simulink model "et_robocon_dev_guy_arch"  (R2013b)
settings: Solver=FixedStepDiscrete  SolverMode=SingleTasking  StartTime=0.0  StopTime=inf  FixedStep=balancer_ts  RelTol=1e-3
undefined symbols (not defined in the file): a_d, a_r, balancerStates_Bus0, Batt, battery_gain, battery_offset, cmd_max, current_mode_status, current_task_operation_status, DiscIntNeverNeededParam, exec_period, Init_Bus0, K, k_f, k_i, k_phidot, k_thetadot, lightCalib, phi_des, R, STATE, TRACK_MODE_LIST, ts2, W
libraries: legonxtlib x34, simulink x19, simulink_extras x4
(part 2 of 5)

== system et_robocon_dev_guy_arch/Main Controller/normal_operation_modes.line_tracking_after_seesaw/line_tracking_mode.tail_controller ==
  note: Could be improved, PI for example
  current : Inport  OutDataTypeStr=single  PortDimensions=1
  desired : Inport  Port=2  OutDataTypeStr=single  PortDimensions=1
  f : TriggerPort  TriggerType=function-call
      settings: CopyFcn=Stateflow.SLINSF.SimulinkMan.removeBlockPreDeleteFcn  PreDeleteFcn=Stateflow.SLINSF.SimulinkMan.unsafePredeleteFcn
  Gain : Gain  Gain=250
  Saturation : Saturate  UpperLimit=100  LowerLimit=-100  OutDataTypeStr=single
  Sum : Sum  Inputs=|+-
  cmd : Outport  OutDataTypeStr=single  PortDimensions=1  InitialOutput=0
  wires:
  Sum/1 -> Gain/1
  current/1 -> Sum/2
  desired/1 -> Sum/1
  Gain/1 -> Saturation/1
  Saturation/1 -> cmd/1

== system et_robocon_dev_guy_arch/Main Controller/normal_operation_modes.line_tracking_after_seesaw/line_tracking_mode.turnLightOn ==
  f : TriggerPort  TriggerType=function-call
      settings: CopyFcn=Stateflow.SLINSF.SimulinkMan.removeBlockPreDeleteFcn  PreDeleteFcn=Stateflow.SLINSF.SimulinkMan.unsafePredeleteFcn
  Light Sensor Switch ON : S-Function  FunctionName=sfun_light_sw  Parameters=-1,ip,sw  EnableBusSupport=off  mask(Light Sensor ON/OFF Switch){ip=S3, sw=ON}
      mask prompts: ip "port:"; sw "switch"
      mask help: LEGO Mindstorms NXT Light Sensor switch.
      mask init:
      | [data, map]=imread('LIGHT_SENSOR.gif');
      | pic=ind2rgb(data,map);
      mask TypeOptions ip: S1 | S2 | S3 | S4
      mask TypeOptions sw: ON | OFF
      mask Display:
      | image(pic)
      | color('red')
      | fprintf('%s, %s',ip,sw)

== system et_robocon_dev_guy_arch/Main Controller/normal_operation_modes.line_tracking_mode/line_tracking_mode.Speak ==
  f : TriggerPort  TriggerType=function-call
      settings: CopyFcn=Stateflow.SLINSF.SimulinkMan.removeBlockPreDeleteFcn  PreDeleteFcn=Stateflow.SLINSF.SimulinkMan.unsafePredeleteFcn
  Constant : Constant  Value=50
  Speaker : legonxtlib/Speaker  sinputMode=Volume only  sspeakerFreq=800  sspeakerVolume=50  sspeakerDuration=100
  wires:
  Constant/1 -> Speaker/1

== system et_robocon_dev_guy_arch/Main Controller/normal_operation_modes.line_tracking_mode/line_tracking_mode.Track.analyzeEncoders ==
  rawSensors : Inport  OutDataTypeStr=Bus: Sensors_Bus  PortDimensions=1
  f : TriggerPort  TriggerType=function-call
      settings: CopyFcn=Stateflow.SLINSF.SimulinkMan.removeBlockPreDeleteFcn  PreDeleteFcn=Stateflow.SLINSF.SimulinkMan.unsafePredeleteFcn
  AngleCounter : Subsystem
  Bus Creator : BusCreator  Inputs=2
  Bus Selector : BusSelector  OutputSignals=theta_R,theta_L
  Signal Conversion : SignalConversion
  Signal Conversion1 : SignalConversion
  AngleCount : Outport  OutDataTypeStr=uint8  PortDimensions=1  InitialOutput=0
  EncoderReset : Outport  Port=2  OutDataTypeStr=single  PortDimensions=1  InitialOutput=0
  Angle : Outport  Port=3  OutDataTypeStr=single  PortDimensions=1  InitialOutput=0
  Distance : Outport  Port=4  OutDataTypeStr=single  PortDimensions=1  InitialOutput=0
  wires:
  rawSensors/1 -> Bus Selector/1
  Bus Creator/1 -> AngleCounter/1(EC)
  Bus Selector/1 -> Signal Conversion/1  "<theta_R>"
  Bus Selector/2 -> Signal Conversion1/1  "<theta_L>"
  Signal Conversion/1 -> Bus Creator/1  "R"
  Signal Conversion1/1 -> Bus Creator/2  "L"
  AngleCounter/1(AngleCount) -> AngleCount/1
  AngleCounter/2(EncoderReseted) -> EncoderReset/1
  AngleCounter/3(Angle) -> Angle/1
  AngleCounter/4(Distance) -> Distance/1

== system et_robocon_dev_guy_arch/Main Controller/normal_operation_modes.line_tracking_mode/line_tracking_mode.Track.lineTracker ==
  lightSignal : Inport  OutDataTypeStr=single  PortDimensions=1
  flagSteering : Inport  Port=2  OutDataTypeStr=single  PortDimensions=1
  PID : Inport  Port=3  OutDataTypeStr=single  PortDimensions=5
  fwd : Inport  Port=4  OutDataTypeStr=single  PortDimensions=1
  f : TriggerPort  TriggerType=function-call
      settings: CopyFcn=Stateflow.SLINSF.SimulinkMan.removeBlockPreDeleteFcn  PreDeleteFcn=Stateflow.SLINSF.SimulinkMan.unsafePredeleteFcn
  Gain : Gain  Gain=100
  Handler : Subsystem
  LCD : legonxtlib/LCD  slcdStr=PID  slcdLine=6  slcdFormat=Decimal
  Signal Conversion : SignalConversion
  SwitchForFreeSteering : Subsystem
  cmd : Outport  InitialOutput=[0 0]
  wires:
  Handler/1(cmd) -> Signal Conversion/1
  lightSignal/1 -> SwitchForFreeSteering/3(LightSens)
  SwitchForFreeSteering/1(Steering) -> Gain/1, Handler/1(steering)
  flagSteering/1 -> SwitchForFreeSteering/1(FlagSteering)
  PID/1 -> SwitchForFreeSteering/2(PID)
  fwd/1 -> Handler/2(fwd)
  Signal Conversion/1 -> cmd/1
  Gain/1 -> LCD/1

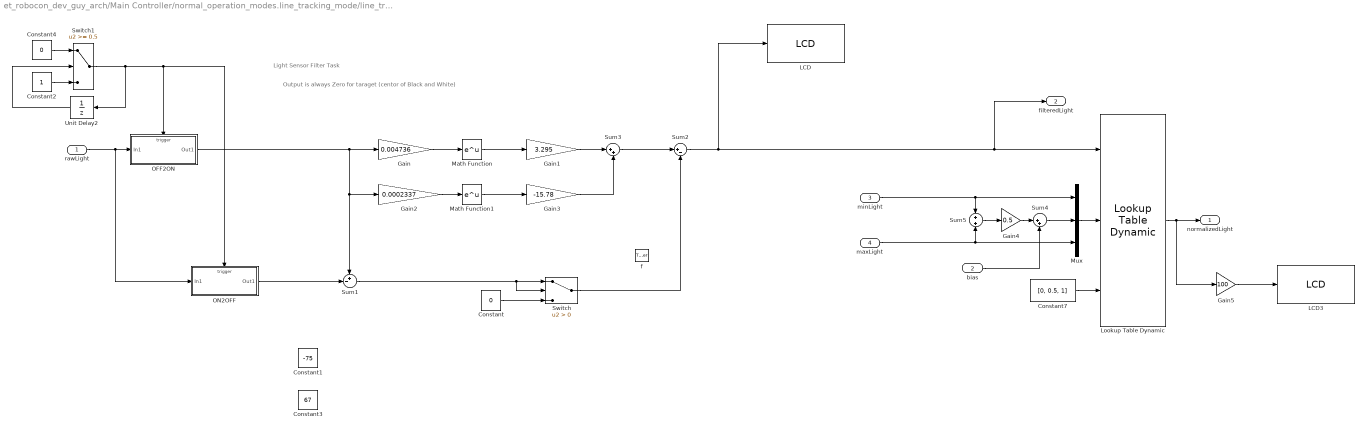
== system et_robocon_dev_guy_arch/Main Controller/normal_operation_modes.line_tracking_mode/line_tracking_mode.Track.processLight ==
  note: Output is always Zero for taraget (centor of Black and White)
  note: Light Sensor Filter Task
  rawLight : Inport  OutDataTypeStr=single  PortDimensions=1
  bias : Inport  Port=2  OutDataTypeStr=single  PortDimensions=1
  minLight : Inport  Port=3  OutDataTypeStr=single  PortDimensions=1
  maxLight : Inport  Port=4  OutDataTypeStr=single  PortDimensions=1
  f : TriggerPort  TriggerType=function-call
      settings: CopyFcn=Stateflow.SLINSF.SimulinkMan.removeBlockPreDeleteFcn  PreDeleteFcn=Stateflow.SLINSF.SimulinkMan.unsafePredeleteFcn
  Constant : Constant  Value=0  OutDataTypeStr=single  SampleTime=-1
  Constant1 : Constant  Value=-75  OutDataTypeStr=single  SampleTime=-1
  Constant2 : Constant  OutDataTypeStr=uint8
  Constant3 : Constant  Value=67  OutDataTypeStr=single  SampleTime=-1
  Constant4 : Constant  Value=0  OutDataTypeStr=uint8
  Constant7 : Constant  Value=[0, 0.5, 1]  OutDataTypeStr=single  SampleTime=-1
  Gain : Gain  Gain=0.004736
  Gain1 : Gain  Gain=3.295
  Gain2 : Gain  Gain=0.0002337
  Gain3 : Gain  Gain=-15.78
  Gain4 : Gain  Gain=0.5
  Gain5 : Gain  Gain=100
  LCD : legonxtlib/LCD  slcdStr=L  slcdLine=4  slcdFormat=Decimal
  LCD3 : legonxtlib/LCD  slcdStr=N  slcdLine=5  slcdFormat=Decimal
  Lookup Table Dynamic : simulink/Lookup Tables/Lookup Table Dynamic  LookUpMeth=Interpolation-Use End Values  OutDataTypeStr=fixdt('single')  OutputDataTypeScalingMode=Specify via dialog  OutDataType=fixdt('single')  OutScaling=[]  RndMeth=Simplest  DoSatur=off
  Math Function : Math  SaturateOnIntegerOverflow=on
  Math Function1 : Math  SaturateOnIntegerOverflow=on
  Mux : Mux  Inputs=3
  OFF2ON : Subsystem  TreatAsAtomicUnit=on
  ON2OFF : Subsystem  TreatAsAtomicUnit=on
  Sum1 : Sum  Inputs=+-|
  Sum2 : Sum  Inputs=|+-
  Sum3 : Sum  Inputs=|++
  Sum4 : Sum  Inputs=|++  OutDataTypeStr=single  RndMeth=Simplest
  Sum5 : Sum  Inputs=+|+
  Switch : Switch  Criteria=u2 > Threshold  RndMeth=Simplest
  Switch1 : Switch  Threshold=0.5
  Unit Delay2 : UnitDelay  SampleTime=-1
  normalizedLight : Outport  OutDataTypeStr=single  PortDimensions=1  InitialOutput=0
  filteredLight : Outport  Port=2  OutDataTypeStr=single  PortDimensions=1  InitialOutput=0
  wires:
  minLight/1 -> Sum5/1, Mux/1
  Mux/1 -> Lookup Table Dynamic/2
  Sum4/1 -> Mux/2
  Sum5/1 -> Gain4/1
  bias/1 -> Sum4/2
  Constant7/1 -> Lookup Table Dynamic/3
  Lookup Table Dynamic/1 -> Gain5/1, normalizedLight/1
  Sum2/1 -> filteredLight/1, Lookup Table Dynamic/1, LCD/1
  Switch/1 -> Sum2/2
  Sum3/1 -> Sum2/1
  Gain3/1 -> Sum3/2
  Gain1/1 -> Sum3/1
  Math Function1/1 -> Gain3/1
  Gain2/1 -> Math Function1/1
  Sum1/1 -> Switch/2, Switch/1
  Constant/1 -> Switch/3
  Math Function/1 -> Gain1/1
  Gain/1 -> Math Function/1
  OFF2ON/1(Out1) -> Gain2/1, Sum1/1, Gain/1
  ON2OFF/1(Out1) -> Sum1/2
  Unit Delay2/1 -> Switch1/2
  Constant4/1 -> Switch1/1
  Constant2/1 -> Switch1/3
  Switch1/1 -> Unit Delay2/1, OFF2ON/Trigger, ON2OFF/Trigger
  rawLight/1 -> ON2OFF/1(In1), OFF2ON/1(In1)
  Gain4/1 -> Sum4/1
  maxLight/1 -> Sum5/2, Mux/3
  Gain5/1 -> LCD3/1

== system et_robocon_dev_guy_arch/Main Controller/normal_operation_modes.line_tracking_mode/line_tracking_mode.balanceControl ==
  rawSensors : Inport  OutDataTypeStr=Bus: Sensors_Bus  PortDimensions=1
  lineTrackCmd : Inport  Port=2  OutDataTypeStr=single  PortDimensions=2
  gyroTrick : Inport  Port=3  OutDataTypeStr=single  PortDimensions=1
  f : TriggerPort  TriggerType=function-call
      settings: CopyFcn=Stateflow.SLINSF.SimulinkMan.removeBlockPreDeleteFcn  PreDeleteFcn=Stateflow.SLINSF.SimulinkMan.unsafePredeleteFcn
  Bus Selector : BusSelector  OutputSignals=gyro,theta_L,theta_R,battery
  Constant3 : Constant  Value=600  OutDataTypeStr=uint16
  Data Type Conversion2 : DataTypeConversion  OutDataTypeStr=single  RndMeth=Simplest
      settings: AttributesFormatString=Round = %<RndMeth>
  Demux : Demux  Outputs=2
  ForSimulation : Subsystem  TreatAsAtomicUnit=on  RTWFcnName=balance_control  RTWFileName=balancer
      settings: RTWFcnNameOpts=User specified  RTWFileNameOpts=User specified  FunctionWithSeparateData=on
  Low Pass Filter : Subsystem
  Sum : Sum
  leftPWM : Outport  OutDataTypeStr=single  PortDimensions=1
  rightPWM : Outport  Port=2
  wires:
  ForSimulation/1(pwm_l) -> rightPWM/1
  ForSimulation/2(pwm_r) -> leftPWM/1
  rawSensors/1 -> Bus Selector/1
  lineTrackCmd/1 -> Demux/1
  Bus Selector/2 -> ForSimulation/5(theta_m_l)  "<theta_L>"
  Bus Selector/3 -> ForSimulation/6(theta_m_r)  "<theta_R>"
  Bus Selector/1 -> ForSimulation/3(gyro)  "<gyro>"
  Bus Selector/4 -> Low Pass Filter/1(u)  "<battery>"
  Low Pass Filter/1(y) -> ForSimulation/7(battery)
  Demux/1 -> ForSimulation/1(cmd_forward)
  Demux/2 -> ForSimulation/2(cmd_turn)
  Constant3/1 -> Data Type Conversion2/1
  Data Type Conversion2/1 -> Sum/1  "gyro_offset"
  gyroTrick/1 -> Sum/2
  Sum/1 -> ForSimulation/4(gyro_offset)

== system et_robocon_dev_guy_arch/Main Controller/normal_operation_modes.line_tracking_mode/line_tracking_mode.phiController ==
  phi : Inport  OutDataTypeStr=single  PortDimensions=1
  desiredPhi : Inport  Port=2  OutDataTypeStr=single  PortDimensions=1
  battery : Inport  Port=3  OutDataTypeStr=double  PortDimensions=1
  f : TriggerPort  TriggerType=function-call
      settings: CopyFcn=Stateflow.SLINSF.SimulinkMan.removeBlockPreDeleteFcn  PreDeleteFcn=Stateflow.SLINSF.SimulinkMan.unsafePredeleteFcn
  Divide : Product  Inputs=*/
  Gain : Gain  Gain=-10
  Gain1 : Gain  Gain=100
  Saturation1 : Saturate  UpperLimit=100  LowerLimit=-100  OutDataTypeStr=single
  Sum : Sum  Inputs=|+-
  cmd : Outport
  wires:
  Saturation1/1 -> cmd/1
  Gain/1 -> Divide/1
  Divide/1 -> Gain1/1
  Gain1/1 -> Saturation1/1
  battery/1 -> Divide/2
  Sum/1 -> Gain/1
  phi/1 -> Sum/2
  desiredPhi/1 -> Sum/1

== system et_robocon_dev_guy_arch/Main Controller/normal_operation_modes.line_tracking_mode/line_tracking_mode.tail_controller ==
  note: Could be improved, PI for example
  current : Inport  OutDataTypeStr=single  PortDimensions=1
  desired : Inport  Port=2  OutDataTypeStr=single  PortDimensions=1
  f : TriggerPort  TriggerType=function-call
      settings: CopyFcn=Stateflow.SLINSF.SimulinkMan.removeBlockPreDeleteFcn  PreDeleteFcn=Stateflow.SLINSF.SimulinkMan.unsafePredeleteFcn
  Gain : Gain  Gain=250
  Saturation : Saturate  UpperLimit=100  LowerLimit=-100  OutDataTypeStr=single
  Sum : Sum  Inputs=|+-
  cmd : Outport  OutDataTypeStr=single  PortDimensions=1  InitialOutput=0
  wires:
  Sum/1 -> Gain/1
  current/1 -> Sum/2
  desired/1 -> Sum/1
  Gain/1 -> Saturation/1
  Saturation/1 -> cmd/1

== system et_robocon_dev_guy_arch/Main Controller/normal_operation_modes.line_tracking_mode/line_tracking_mode.turnLightOn ==
  f : TriggerPort  TriggerType=function-call
      settings: CopyFcn=Stateflow.SLINSF.SimulinkMan.removeBlockPreDeleteFcn  PreDeleteFcn=Stateflow.SLINSF.SimulinkMan.unsafePredeleteFcn
  Light Sensor Switch ON : S-Function  FunctionName=sfun_light_sw  Parameters=-1,ip,sw  EnableBusSupport=off  mask(Light Sensor ON/OFF Switch){ip=S3, sw=ON}
      mask prompts: ip "port:"; sw "switch"
      mask help: LEGO Mindstorms NXT Light Sensor switch.
      mask init:
      | [data, map]=imread('LIGHT_SENSOR.gif');
      | pic=ind2rgb(data,map);
      mask TypeOptions ip: S1 | S2 | S3 | S4
      mask TypeOptions sw: ON | OFF
      mask Display:
      | image(pic)
      | color('red')
      | fprintf('%s, %s',ip,sw)

== system et_robocon_dev_guy_arch/Main Controller/normal_operation_modes.see_saw_mario/see_saw_mode.Speak ==
  f : TriggerPort  TriggerType=function-call
      settings: CopyFcn=Stateflow.SLINSF.SimulinkMan.removeBlockPreDeleteFcn  PreDeleteFcn=Stateflow.SLINSF.SimulinkMan.unsafePredeleteFcn
  Constant : Constant  Value=50
  Speaker : legonxtlib/Speaker  sinputMode=Volume only  sspeakerFreq=800  sspeakerVolume=50  sspeakerDuration=100
  wires:
  Constant/1 -> Speaker/1

== stateflow chart et_robocon_dev_guy_arch/State Estimation/StateEstimation/Reset Subsystem ==
  state CheckForReset
    bind: doProcess;
    entry: doProcess;
    during: doProcess;
  (default) -> CheckForReset
  CheckForReset -> CheckForReset : [init_flag == 1]
  data: init_flag input
  events: doProcess output FUNCTION_CALL_EVENT

== stateflow chart et_robocon_dev_guy_arch/Main Controller/normal_operation_modes.see_saw_mario ==
  state see_saw_mode
    entry:
    des_vel = single(0.1);
    desired_tail = single(0);
    BT_status_out = single(1);
    during:
    normalizedLight = processLight(sensors.light,lightCalib);
    PWM.tail = tail_controller(sensors.theta_T, desired_tail);
    state StandUp
      entry:
      debugFlag = uint16(602);
      initFlags.theta = single(1);
      initFlags.gyroReset = single(1);
    state light = processLight(rawLight,lightCalib) [function]
    state Balancing
      state SeesawLogic [parallel]
        settings: executionOrder=1
        state StationnaryBalance
          entry:
          Speak;
          debugFlag = uint16(603);
          initFlags.theta = single(0);
          initFlags.gyroReset = single(0);
          desired_states = balancerStates_Bus0;
        state ApproachToSeeSaw
          entry: debugFlag = uint16(604);
          during:
          turningPWM = phiController(states.phi,desired_phi, sensors.battery)+...
          lineTracker(single(-0.1), normalizedLight, single(1.3), sensors.battery);
          exit:
          turningPWM = single(0);
        state Seesaw
          state ControlledGoingUp
            entry:
            phi0 = states.phi;
            desired_phi = phi0;
            exit: turningPWM = single(0);
            state JumpOnIt
              entry:
              Speak;
              debugFlag = uint16(606);
              theta_ref = states.balancerStates.theta;
              des_vel = single(0.15);
              du: turningPWM = phiController(states.phi,desired_phi, sensors.battery);
            state GoingUP
              entry:
              debugFlag = uint16(607);
              des_vel = single(0.1);
              during:
              turningPWM = phiController(states.phi,desired_phi, sensors.battery)+...
              single(3)*lineTracker(single(0.15), normalizedLight, single(1), sensors.battery);
              exit:
              des_vel = single(0);
            state WaitForPrincess
              entry:
              debugFlag = uint16(608);
              BT_status_out = single(2);
              du:
              turningPWM = phiController(states.phi,desired_phi,sensors.battery);
            (default) -> JumpOnIt
            JumpOnIt -> GoingUP : [states.balancerStates.theta >= theta_ref+single(1.6)]
            GoingUP -> WaitForPrincess : [states.balancerStates.theta >= theta_ref + single(18)]
          state GoingDown
            during:
            turningPWM = single(-1.3)*lineTracker(single(0.7), normalizedLight, single(1.2), sensors.battery)+...
            single(1)*phiController(states.phi,desired_phi,sensors.battery);
            state GoingBack
              entry:
              debugFlag = uint16(609);
              des_vel = single(-0.06);
              exit:
              des_vel = single(-0.06);
            state WaitForPrincess2
              entry:
              debugFlag = uint16(610);
              BT_status_out = single(3);
              %during:turningPWM = phiController(states.phi,desired_phi,sensors.battery);
            state GetOff
              entry:
              debugFlag = uint16(611);
              des_vel = single(-0.1);
            (default) -> GoingBack
            GoingBack -> WaitForPrincess2 : [states.balancerStates.theta <= theta_ref + single(12)]
            WaitForPrincess2 -> GetOff : [sensors.BT_status_in == single(103)]
          state GetOff1
            entry:
            debugFlag = uint16(6112);
            des_vel = single(-0.08);
            du:
            turningPWM = phiController(states.phi,desired_phi+single(0.05),sensors.battery);
          state FindingLine
            en:
            turningPWM = phiController(states.phi,desired_phi,sensors.battery);
            des_vel = single(0);
            state TurnAndBackup
              entry:
              debugFlag = uint16(612);
              BT_status_out = single(4);
              du:
              desired_phi = desired_phi - single(0.003);
              des_vel = single(0);
              turningPWM = phiController(states.phi,desired_phi,sensors.battery);
            state HuntLine
              entry: debugFlag = uint16(613)
              desired_phi = states.phi;
              theta_ref_2 = states.balancerStates.theta;
              du: turningPWM = phiController(states.phi,desired_phi,sensors.battery);
              state GoForward
                en:  des_vel= single(0.04);
                entry: debugFlag = uint16(6131);
              state BackUpB
                en: des_vel = single(-0.04)
                entry: debugFlag = uint16(6132);
              BackUpB -> GoForward : [states.balancerStates.theta <= theta_ref_2 - single(3) ]
              (default) -> BackUpB
              GoForward -> BackUpB : [states.balancerStates.theta >= theta_ref_2 + single(3) ]
            state TurnAndBackup1
              entry:
              Speak
              debugFlag = uint16(614);
              des_vel = des_vel / single(3);
              du:
              desired_phi = desired_phi - single(0.003);
              turningPWM = phiController(states.phi,desired_phi,sensors.battery);
            state GoForwardUntilLine
              en:
              Speak;
              debugFlag = uint16(615)
              des_vel = single(0);
            (default) -> TurnAndBackup
            TurnAndBackup -> HuntLine : [phi0-states.phi > single(1.6)]
            HuntLine -> TurnAndBackup1 : [normalizedLight >= single(0.5)]
            TurnAndBackup1 -> GoForwardUntilLine : [phi0-states.phi > single(2.3)]
          (default) -> ControlledGoingUp
          WaitForPrincess -> GoingDown : [sensors.BT_status_in == single(102)]
          GoingDown -> GetOff1 : [states.balancerStates.theta <= theta_ref ]
          GetOff1 -> FindingLine : [states.balancerStates.theta <= theta_ref - single(5)]
        state RaceDone
          entry: debugFlag = uint16(599);
          BT_status_out = single(5);
          current_mode_status = OperationModeStatusEnum.SUCCESSFULLY_COMPLETED;
        (default) -> StationnaryBalance
        StationnaryBalance -> ApproachToSeeSaw
        ApproachToSeeSaw -> Seesaw : [states.balancerStates.theta_dot < single(1)]
        GoForwardUntilLine -> RaceDone : after(1,sec)
      state After [parallel]
        during:
        forwardPWM = balance_ctrl(states.balancerStates, des_vel ,sensors.battery)
        PWM.left = forwardPWM + turningPWM;
        PWM.right = forwardPWM - turningPWM;
        settings: executionOrder=2
    state cmd = phiController(phi,desiredPhi,battery) [function]
    state cmd = lineTracker(desiredLight,light,trackingPower,battery) [function]
    state Speak [function]
    state cmd = tail_controller(current,desired) [function]
    state cmd = balance_ctrl(balancerStates,desired_velocity,battery) [function]
    (default) -> StandUp
    StandUp -> Balancing
  data: rawLight function_input single size=1; lightCalib function_input Bus: Light_Bus size=1; light function_output; cmd function_output; phi function_input single size=1; desiredPhi function_input single size=1; battery function_input double size=1; cmd function_output single size=1; desiredLight function_input single size=1; light function_input single size=1; trackingPower function_input single size=1; battery function_input double size=1; current function_input single size=1; desired function_input single size=1; cmd function_output single size=1; balancerStates function_input Bus: Balancer_States_Bus size=1; desired_velocity function_input single size=1; battery function_input double size=1; cmd function_output single size=1; states input Bus: States_Bus size=1; sensors input Bus: Sensors_Bus size=1; PWM output Bus: PWM_bus size=1; initFlags output Bus: Init_Bus size=1; debugFlag output uint16 size=1; desired_states local Bus: Balancer_States_Bus size=1; desired_tail local single size=1; current_mode_status data_store_memory; balancerStates_Bus0 parameter Bus: Balancer_States_Bus size=1; lightCalib data_store_memory; normalizedLight local single size=1; des_vel local single size=1; theta_ref local single size=1; forwardPWM local single size=1; turningPWM local single size=1; BT_status_out output single size=1; desired_phi local single size=1; phi0 local single size=1; theta_ref_2 local

== stateflow chart et_robocon_dev_guy_arch/Main Controller/normal_operation_modes.light_calibration_up ==
  state wait
    entry:debugFlag = uint16(200);
  state MoveUp
    entry:debugFlag = uint16(201);
    PWM.tail = single(-50);
  state Reset
    entry:debugFlag = uint16(202);
    PWM.tail = single(0);
    initFlags.tail = single(1);
    exit:
    initFlags.tail = single(0);
    desired_tail = single(0);
  state light_sensor_calibration_up
    %during, exit: PWM.tail = tail_controller(sensors.theta_T,single(1.6))
    state WaitForBlack
      entry: debugFlag = uint16(310);
    state StoreBlack
      entry: lightCalib.black = sensors.light;
      debugFlag = uint16(311);
    state WaitForWhite
      entry: debugFlag = uint16(312)
    state StoreWhite
      entry: lightCalib.white = sensors.light;
      debugFlag = uint16(313);
    state CalibComplete
      entry:
      debugFlag = uint16(318);
      current_task_operation_status = OperationModeStatusEnum.SUCCESSFULLY_COMPLETED;
    state cmd = tail_controller(current,desired) [function]
    (default) -> WaitForBlack
    WaitForBlack -> StoreBlack : [hasChangedFrom(touch,single(0))]
    StoreBlack -> WaitForWhite : after(0.2,sec){Speak;}
    WaitForWhite -> StoreWhite : [hasChangedFrom(touch,single(0))]
    StoreWhite -> CalibComplete : after(0.2,sec){Speak;}
  state Speak [function]
  (default) -> wait
  wait -> MoveUp : [hasChangedFrom(touch,single(0))]{Speak;}
  MoveUp -> Reset : after(2,sec)
  Reset -> light_sensor_calibration_up : after(1,sec){Speak;}
  data: current function_input single size=1; desired function_input single size=1; cmd function_output single size=1; sensors input Bus: Sensors_Bus size=1; lightCalib data_store_memory; current_task_operation_status data_store_memory; debugFlag output uint16; touch input single size=1; PWM output Bus: PWM_bus size=1; initFlags output Bus: Init_Bus size=1; desired_tail local

== stateflow chart et_robocon_dev_guy_arch/Main Controller/normal_operation_modes.light_calibration_up_flashing_on_map ==
  state LightSensorCalibFlashing
    during:
    on every(3, tick): filteredLight = processLight(sensors.light);
    state WaitForBlack
      entry: debugFlag = uint16(310);
    state StoreBlack
      entry: lightCalib.flashingMapBlack = filteredLight;
      debugFlag = uint16(311);
      Speak;
    state WaitForWhite
      entry: debugFlag = uint16(312);
      Speak;
    state StoreWhite
      entry: lightCalib.flashingMapWhite = filteredLight;
      debugFlag = uint16(313);
      Speak;
      exit:
      turnLightOn;
      Speak;
    state CalibComplete
      entry:
      debugFlag = uint16(318);
      current_task_operation_status = OperationModeStatusEnum.SUCCESSFULLY_COMPLETED;
    state cmd = tail_controller(current,desired) [function]
    state Speak [function]
    state turnLightOn [function]
    state filteredLight  = processLight(rawLight) [function]
    (default) -> WaitForBlack
    WaitForBlack -> StoreBlack : [hasChangedFrom(touch,single(0))]
    StoreBlack -> WaitForWhite : after(1,sec)
    WaitForWhite -> StoreWhite : [hasChangedFrom(touch,single(0))]
    StoreWhite -> CalibComplete : after(1,sec)
  data: current function_input single size=1; desired function_input single size=1; cmd function_output single size=1; rawLight function_input single size=1; filteredLight function_output single size=1; sensors input Bus: Sensors_Bus size=1; lightCalib data_store_memory; current_task_operation_status data_store_memory; debugFlag output uint16; touch input single size=1; filteredLight local

== system et_robocon_dev_guy_arch/Main Controller/normal_operation_modes.see_saw_mario/see_saw_mode.balance_ctrl ==
  balancerStates : Inport  OutDataTypeStr=Bus: Balancer_States_Bus  PortDimensions=1
  desired_velocity : Inport  Port=2  OutDataTypeStr=single  PortDimensions=1  BusOutputAsStruct=on
  battery : Inport  Port=3  OutDataTypeStr=double  PortDimensions=1
  f : TriggerPort  TriggerType=function-call
      settings: CopyFcn=Stateflow.SLINSF.SimulinkMan.removeBlockPreDeleteFcn  PreDeleteFcn=Stateflow.SLINSF.SimulinkMan.unsafePredeleteFcn
  Bus to Vector : BusToVector
  Constant : Constant  Value=0  OutDataTypeStr=single
  Constant1 : Constant  Value=0  OutDataTypeStr=single
  Discrete-Time Integrator : DiscreteIntegrator  SampleTime=-1  ICPrevOutput=DiscIntNeverNeededParam  ICPrevScaledInput=DiscIntNeverNeededParam
  Discrete-Time Integrator1 : DiscreteIntegrator  SampleTime=-1  ICPrevOutput=DiscIntNeverNeededParam  ICPrevScaledInput=DiscIntNeverNeededParam
  Divide : Product  Inputs=*/
  Gain : Gain  Gain=100
  Gain1 : Gain  Gain=K  Multiplication=Matrix(K*u)
  LPF : DiscreteFilter  Numerator=[0.15]  Denominator=[1 -0.85]
  Reshape : Reshape  OutputDimensionality=Column vector (2-D)
  Saturation : Saturate  UpperLimit=100  LowerLimit=-100  OutDataTypeStr=single
  Signal Conversion1 : SignalConversion  ConversionOutput=Virtual bus
  Sum1 : Sum  Inputs=|+-
  Vector Concatenate : Concatenate  NumInputs=5
  m/s --> rad/s : Gain  Gain=1/R
  cmd : Outport  OutDataTypeStr=single  PortDimensions=1  InitialOutput=0
  wires:
  Discrete-Time Integrator1/1 -> Vector Concatenate/5
  Discrete-Time Integrator/1 -> Vector Concatenate/1, Discrete-Time Integrator1/1
  Constant1/1 -> Vector Concatenate/4
  LPF/1 -> Vector Concatenate/3, Discrete-Time Integrator/1
  Constant/1 -> Vector Concatenate/2
  m/s --> rad/s/1 -> LPF/1
  Signal Conversion1/1 -> Bus to Vector/1
  Divide/1 -> Gain/1
  Gain/1 -> Saturation/1
  Gain1/1 -> Divide/1
  Saturation/1 -> cmd/1
  battery/1 -> Divide/2
  Vector Concatenate/1 -> Sum1/1
  balancerStates/1 -> Signal Conversion1/1
  Bus to Vector/1 -> Sum1/2
  desired_velocity/1 -> m/s --> rad/s/1
  Sum1/1 -> Reshape/1
  Reshape/1 -> Gain1/1

== system et_robocon_dev_guy_arch/Main Controller/normal_operation_modes.see_saw_mario/see_saw_mode.lineTracker ==
  desiredLight : Inport  OutDataTypeStr=single  PortDimensions=1
  light : Inport  Port=2  OutDataTypeStr=single  PortDimensions=1
  trackingPower : Inport  Port=3  OutDataTypeStr=single  PortDimensions=1
  battery : Inport  Port=4  OutDataTypeStr=double  PortDimensions=1
  f : TriggerPort  TriggerType=function-call
      settings: CopyFcn=Stateflow.SLINSF.SimulinkMan.removeBlockPreDeleteFcn  PreDeleteFcn=Stateflow.SLINSF.SimulinkMan.unsafePredeleteFcn
  Constant : Constant  Value=0  OutDataTypeStr=single
  Dead Zone : DeadZone  LowerValue=-0.02  UpperValue=0.02  SaturateOnIntegerOverflow=on
  Divide : Product  Inputs=*/
  Gain : Gain  Gain=100
  LPF and deriv : Subsystem
  PD : Gain  Gain="[4  0.02]/2"  Multiplication=Matrix(K*u)
  Product : Product
  Saturation : Saturate  UpperLimit=6  LowerLimit=-6
  Saturation1 : Saturate  UpperLimit=100  LowerLimit=-100  OutDataTypeStr=single
  Sum : Sum  Inputs=|+-
  Vector Concatenate : Concatenate
  Vector Concatenate1 : Concatenate
  switch side of line : Gain  Gain=-1
  cmd : Outport  OutDataTypeStr=single  PortDimensions=1
  wires:
  Divide/1 -> Gain/1
  Gain/1 -> Saturation1/1
  battery/1 -> Divide/2
  Saturation1/1 -> switch side of line/1
  Product/1 -> Divide/1
  trackingPower/1 -> Product/1
  Saturation/1 -> Product/2
  PD/1 -> Saturation/1
  Dead Zone/1 -> PD/1
  Sum/1 -> Dead Zone/1
  Vector Concatenate1/1 -> Sum/2
  Vector Concatenate/1 -> Sum/1
  light/1 -> Vector Concatenate1/1, LPF and deriv/1(light)
  LPF and deriv/1(light_dot) -> Vector Concatenate1/2
  Constant/1 -> Vector Concatenate/2  "desired light derivative"
  desiredLight/1 -> Vector Concatenate/1
  switch side of line/1 -> cmd/1

== system et_robocon_dev_guy_arch/Main Controller/normal_operation_modes.see_saw_mario/see_saw_mode.phiController ==
  phi : Inport  OutDataTypeStr=single  PortDimensions=1
  desiredPhi : Inport  Port=2  OutDataTypeStr=single  PortDimensions=1
  battery : Inport  Port=3  OutDataTypeStr=double  PortDimensions=1
  f : TriggerPort  TriggerType=function-call
      settings: CopyFcn=Stateflow.SLINSF.SimulinkMan.removeBlockPreDeleteFcn  PreDeleteFcn=Stateflow.SLINSF.SimulinkMan.unsafePredeleteFcn
  Divide : Product  Inputs=*/
  Gain : Gain  Gain=-10
  Gain1 : Gain  Gain=100
  Saturation1 : Saturate  UpperLimit=100  LowerLimit=-100  OutDataTypeStr=single
  Sum : Sum  Inputs=|+-
  cmd : Outport
  wires:
  Saturation1/1 -> cmd/1
  Gain/1 -> Divide/1
  Divide/1 -> Gain1/1
  Gain1/1 -> Saturation1/1
  battery/1 -> Divide/2
  Sum/1 -> Gain/1
  phi/1 -> Sum/2
  desiredPhi/1 -> Sum/1

== system et_robocon_dev_guy_arch/Main Controller/normal_operation_modes.see_saw_mario/see_saw_mode.processLight ==
  rawLight : Inport  OutDataTypeStr=single  PortDimensions=1
  lightCalib : Inport  Port=2  OutDataTypeStr=Bus: Light_Bus  PortDimensions=1
  f : TriggerPort  TriggerType=function-call
      settings: CopyFcn=Stateflow.SLINSF.SimulinkMan.removeBlockPreDeleteFcn  PreDeleteFcn=Stateflow.SLINSF.SimulinkMan.unsafePredeleteFcn
  Bus Selector : BusSelector  OutputSignals=black,white
  Gain : Gain  Gain=0.3
  Gain1 : Gain  Gain=1/100
  LCD : legonxtlib/LCD  slcdStr=NLight  slcdLine=5  slcdFormat=Decimal
  Sum : Sum  Inputs=|+-
  Sum1 : Sum  Inputs=|++
  Sum2 : Sum  Inputs=|+-
  light : Outport
  wires:
  Gain1/1 -> light/1  "normalizeLight"
  Sum2/1 -> LCD/1, Gain1/1
  Sum1/1 -> Sum2/2
  rawLight/1 -> Sum2/1
  Gain/1 -> Sum1/1
  Sum/1 -> Gain/1
  Bus Selector/2 -> Sum/2, Sum1/2  "<white>"
  Bus Selector/1 -> Sum/1  "<black>"
  lightCalib/1 -> Bus Selector/1

== system et_robocon_dev_guy_arch/Main Controller/normal_operation_modes.see_saw_mario/see_saw_mode.tail_controller ==
  note: Could be improved, PI for example
  current : Inport  OutDataTypeStr=single  PortDimensions=1
  desired : Inport  Port=2  OutDataTypeStr=single  PortDimensions=1
  f : TriggerPort  TriggerType=function-call
      settings: CopyFcn=Stateflow.SLINSF.SimulinkMan.removeBlockPreDeleteFcn  PreDeleteFcn=Stateflow.SLINSF.SimulinkMan.unsafePredeleteFcn
  Gain : Gain  Gain=250
  Saturation : Saturate  UpperLimit=100  LowerLimit=-100  OutDataTypeStr=single
  Sum : Sum  Inputs=|+-
  cmd : Outport  OutDataTypeStr=single  PortDimensions=1  InitialOutput=0
  wires:
  Saturation/1 -> cmd/1
  Gain/1 -> Saturation/1
  desired/1 -> Sum/1
  current/1 -> Sum/2
  Sum/1 -> Gain/1

== system et_robocon_dev_guy_arch/State Estimation/Data Type Conversion Unit Conversion Tail Initialization ==
  u : Inport
  init_tail : Inport  Port=2
  Bus Creator : BusCreator  Inputs=11  OutDataTypeStr=Bus: Sensors_Bus
  Bus Selector : BusSelector  OutputSignals=theta_L,theta_R,theta_T,light,gyro,sonar,battery,touch,time,ok_button,BT_status_in
  Degrees to Radians{,1..2,4} (4 alike) : simulink_extras/Transformations/Degrees to Radians
  Low Pass Filter : Subsystem
  Process Sonar : Subsystem  Commented=through
  Vmax : Subsystem
  tail processing : Subsystem
  y : Outport
  wires:
  Bus Selector/11 -> Bus Creator/11  "<BT_status_in>"
  Process Sonar/1(sonar) -> Bus Creator/6
  Bus Selector/6 -> Process Sonar/1(sonar_in)  "<sonar>"
  Bus Selector/10 -> Bus Creator/10  "<ok_button>"
  init_tail/1 -> tail processing/2(init_tail)
  Bus Selector/9 -> Bus Creator/9  "<time>"
  Bus Selector/8 -> Bus Creator/8  "<touch>"
  tail processing/1(tail) -> Bus Creator/3  "theta_T"
  Degrees to Radians4/1 -> tail processing/1(sensors)
  Vmax/1(Vmax) -> Bus Creator/7  "battery"
  Degrees to Radians2/1 -> Bus Creator/5  "gyro"
  Bus Selector/3 -> Degrees to Radians4/1  "<theta_T>"
  Bus Selector/7 -> Low Pass Filter/1(u)  "<battery>"
  Bus Selector/5 -> Degrees to Radians2/1  "<gyro>"
  Bus Selector/4 -> Bus Creator/4  "<light>"
  Bus Creator/1 -> y/1
  u/1 -> Bus Selector/1
  Degrees to Radians/1 -> Bus Creator/1  "theta_L"
  Bus Selector/2 -> Degrees to Radians1/1  "<theta_R>"
  Bus Selector/1 -> Degrees to Radians/1  "<theta_L>"
  Low Pass Filter/1(y) -> Vmax/1(Battery)  "battery"
  Degrees to Radians1/1 -> Bus Creator/2  "theta_R"

== system et_robocon_dev_guy_arch/State Estimation/Fall Detection ==
  gyro : Inport
      settings: AttributesFormatString=Output data type: %<OutDataTypeStr>
  reset : Inport  Port=2  OutDataTypeStr=boolean
      settings: AttributesFormatString=Output data type: %<OutDataTypeStr>
  Abs : Abs
  Compare To Constant : simulink/Logic and Bit Operations/Compare To Constant  relop=>  const=1  OutDataTypeStr=boolean
  Terminator : Terminator
  aggregate_fall_detection_comparison : Logic  Operator=OR  OutDataTypeStr=boolean
  boolean_to_integer_conversion : DataTypeConversion  OutDataTypeStr=uint8
      settings: AttributesFormatString=Output data type: %<OutDataTypeStr>
  previous_fall_detection_status : UnitDelay  SampleTime=-1
  reset_output_overrice_switch : MultiPortSwitch  DataPortOrder=Zero-based contiguous  Inputs=2  zeroidx=on  InputSameDT=on
  reset_output_value : Constant  Value=false
  reset_output_value1 : Constant  Value=false  OutDataTypeStr=boolean
  fall_detected : Outport
  wires:
  reset_output_overrice_switch/1 -> Terminator/1, previous_fall_detection_status/1
  reset_output_value/1 -> reset_output_overrice_switch/3
  aggregate_fall_detection_comparison/1 -> reset_output_overrice_switch/2
  boolean_to_integer_conversion/1 -> reset_output_overrice_switch/1
  reset/1 -> boolean_to_integer_conversion/1
  previous_fall_detection_status/1 -> aggregate_fall_detection_comparison/2
  Abs/1 -> Compare To Constant/1
  gyro/1 -> Abs/1
  Compare To Constant/1 -> aggregate_fall_detection_comparison/1
  reset_output_value1/1 -> fall_detected/1

== system et_robocon_dev_guy_arch/State Estimation/Gyro Processing ==
  sensors : Inport
  gyroInit : Inport  Port=2
  gyroReset : Inport  Port=3
  Bus Selector1 : BusSelector  OutputSignals=gyro
  Compute psi : Subsystem
  Gyro initialization : Subsystem  TreatAsAtomicUnit=on
  Reset Subsystem : Stateflow chart  TreatAsAtomicUnit=on
  Sum : Sum  Inputs=-+|
  psi : Outport
  psi_dot : Outport  Port=2
  psi filtered : Outport  Port=3
  wires:
  Compute psi/2(Filtered) -> psi filtered/1
  Reset Subsystem/1(doProcess()) -> Compute psi/Trigger
  gyroReset/1 -> Reset Subsystem/1(init_flag)
  Bus Selector1/1 -> Sum/2, Gyro initialization/1(gyro)  "<gyro>"
  Gyro initialization/1(psi_dot_0) -> Sum/1
  Sum/1 -> psi_dot/1, Compute psi/1(gyro)
  Compute psi/1(psi) -> psi/1
  sensors/1 -> Bus Selector1/1
  gyroInit/1 -> Gyro initialization/Enable

== system et_robocon_dev_guy_arch/State Estimation/StateEstimation ==
  note: Conversion from Raw Sensors to States as described in "NXTway plant model.pdf"
  Sensors : Inport
  psi : Inport  Port=2
  psi_dot : Inport  Port=3
  init theta : Inport  Port=4
  Bus Creator1 : BusCreator  OutDataTypeStr=Bus: States_Bus
  Bus Creator2 : BusCreator  Inputs=5  OutDataTypeStr=Bus: Balancer_States_Bus
  Bus Selector1 : BusSelector  OutputSignals=theta_L,theta_R
  Process theta1 : Subsystem
  Reset Subsystem : Stateflow chart  TreatAsAtomicUnit=on
  states : Outport  OutputWhenDisabled=reset  InitialOutput=0
  wires:
  Process theta1/2(psi_out) -> Bus Creator2/2  "psi"
  Reset Subsystem/1(doProcess()) -> Process theta1/Trigger
  Bus Selector1/2 -> Process theta1/3(theta_r)  "<theta_R>"
  Bus Selector1/1 -> Process theta1/2(theta_l)  "<theta_L>"
  init theta/1 -> Reset Subsystem/1(init_flag)
  Process theta1/1(theta) -> Bus Creator2/1
  Process theta1/3(theta_dot) -> Bus Creator2/3
  Process theta1/4(int_theta) -> Bus Creator2/5
  psi_dot/1 -> Bus Creator2/4  "psi_dot"
  Process theta1/6(phi_dot) -> Bus Creator1/3  "phi_dot"
  Bus Creator2/1 -> Bus Creator1/1  "balancerStates"
  Process theta1/5(phi) -> Bus Creator1/2  "phi"
  Sensors/1 -> Bus Selector1/1
  psi/1 -> Process theta1/1(psi)
  Bus Creator1/1 -> states/1
  Process theta1/7(theta_dot_dot) -> Bus Creator1/4  "theta_dot_dot"

== system et_robocon_dev_guy_arch/Hardware/Receive Bluetooth Status/BluetoothOFF ==
  Constant : Constant  Value=single(0)
  BT_status_in : Outport
  wires:
  Constant/1 -> BT_status_in/1

== system et_robocon_dev_guy_arch/Hardware/Receive Bluetooth Status/BluetoothONMario ==
  Data Type Conversion9 : DataTypeConversion  OutDataTypeStr=single
  Rate Transition2 : RateTransition  OutPortSampleTime=0.004
  Receive via Bluetooth(R) Connection : legonxtlib/Receive via Bluetooth(R) Connection  mailbox=3  dataType=uint8  dataSize=1  sampleTime=0.1
  Terminator : Terminator
  BT_status_in : Outport
  wires:
  Data Type Conversion9/1 -> BT_status_in/1
  Rate Transition2/1 -> Data Type Conversion9/1
  Receive via Bluetooth(R) Connection/1 -> Rate Transition2/1
  Receive via Bluetooth(R) Connection/2 -> Terminator/1

== system et_robocon_dev_guy_arch/Hardware/Receive Bluetooth Status/BluetoothONPrincess ==
  Data Type Conversion9 : DataTypeConversion  OutDataTypeStr=single
  Rate Transition2 : RateTransition  OutPortSampleTime=0.004
  Receive via Bluetooth(R) Connection : legonxtlib/Receive via Bluetooth(R) Connection  mailbox=2  dataType=uint8  dataSize=1  sampleTime=0.1
  Terminator : Terminator
  BT_status_in : Outport
  wires:
  Receive via Bluetooth(R) Connection/2 -> Terminator/1
  Receive via Bluetooth(R) Connection/1 -> Rate Transition2/1
  Rate Transition2/1 -> Data Type Conversion9/1
  Data Type Conversion9/1 -> BT_status_in/1

== system et_robocon_dev_guy_arch/Hardware/Send Bluetooth Status/BluetoothOFF ==
  BT_status_out : Inport
  Terminator : Terminator
  wires:
  BT_status_out/1 -> Terminator/1

== system et_robocon_dev_guy_arch/Hardware/Send Bluetooth Status/BluetoothONMario ==
  BT_status_out : Inport
  Data Type Conversion1 : DataTypeConversion  OutDataTypeStr=uint8
  Rate Transition1 : RateTransition  OutPortSampleTime=0.1
  Send via Bluetooth(R) Connection : legonxtlib/Send via Bluetooth(R) Connection  mailbox=2
  wires:
  BT_status_out/1 -> Rate Transition1/1
  Rate Transition1/1 -> Data Type Conversion1/1
  Data Type Conversion1/1 -> Send via Bluetooth(R) Connection/1

== system et_robocon_dev_guy_arch/Hardware/Send Bluetooth Status/BluetoothONPrincess ==
  BT_status_out : Inport
  Data Type Conversion1 : DataTypeConversion  OutDataTypeStr=uint8
  Rate Transition1 : RateTransition  OutPortSampleTime=0.1
  Send via Bluetooth(R) Connection : legonxtlib/Send via Bluetooth(R) Connection  mailbox=3
  wires:
  Data Type Conversion1/1 -> Send via Bluetooth(R) Connection/1
  Rate Transition1/1 -> Data Type Conversion1/1
  BT_status_out/1 -> Rate Transition1/1

== system et_robocon_dev_guy_arch/Main Controller/normal_operation_modes.light_calibration_up_flashing/LightSensorCalibFlashing.processLight/OFF2ON ==
  In1 : Inport
  Trigger : TriggerPort
  Light Sensor Switch ON : S-Function  FunctionName=sfun_light_sw  Parameters=-1,ip,sw  EnableBusSupport=off  mask(Light Sensor ON/OFF Switch){ip=S3, sw=ON}
      mask prompts: ip "port:"; sw "switch"
      mask help: LEGO Mindstorms NXT Light Sensor switch.
      mask init:
      | [data, map]=imread('LIGHT_SENSOR.gif');
      | pic=ind2rgb(data,map);
      mask TypeOptions ip: S1 | S2 | S3 | S4
      mask TypeOptions sw: ON | OFF
      mask Display:
      | image(pic)
      | color('red')
      | fprintf('%s, %s',ip,sw)
  Out1 : Outport
  wires:
  In1/1 -> Out1/1

== system et_robocon_dev_guy_arch/Main Controller/normal_operation_modes.light_calibration_up_flashing/LightSensorCalibFlashing.processLight/ON2OFF ==
  In1 : Inport
  Trigger : TriggerPort  TriggerType=falling
  Light Sensor Switch OFF : S-Function  FunctionName=sfun_light_sw  Parameters=-1,ip,sw  EnableBusSupport=off  mask(Light Sensor ON/OFF Switch){ip=S3, sw=OFF}
      mask prompts: ip "port:"; sw "switch"
      mask help: LEGO Mindstorms NXT Light Sensor switch.
      mask init:
      | [data, map]=imread('LIGHT_SENSOR.gif');
      | pic=ind2rgb(data,map);
      mask TypeOptions ip: S1 | S2 | S3 | S4
      mask TypeOptions sw: ON | OFF
      mask Display:
      | image(pic)
      | color('red')
      | fprintf('%s, %s',ip,sw)
  Out1 : Outport
  wires:
  In1/1 -> Out1/1

== system et_robocon_dev_guy_arch/Main Controller/normal_operation_modes.light_calibration_up_flashing_on_map/LightSensorCalibFlashing.processLight/OFF2ON ==
  In1 : Inport
  Trigger : TriggerPort
  Light Sensor Switch ON : S-Function  FunctionName=sfun_light_sw  Parameters=-1,ip,sw  EnableBusSupport=off  mask(Light Sensor ON/OFF Switch){ip=S3, sw=ON}
      mask prompts: ip "port:"; sw "switch"
      mask help: LEGO Mindstorms NXT Light Sensor switch.
      mask init:
      | [data, map]=imread('LIGHT_SENSOR.gif');
      | pic=ind2rgb(data,map);
      mask TypeOptions ip: S1 | S2 | S3 | S4
      mask TypeOptions sw: ON | OFF
      mask Display:
      | image(pic)
      | color('red')
      | fprintf('%s, %s',ip,sw)
  Out1 : Outport
  wires:
  In1/1 -> Out1/1

== system et_robocon_dev_guy_arch/Main Controller/normal_operation_modes.light_calibration_up_flashing_on_map/LightSensorCalibFlashing.processLight/ON2OFF ==
  In1 : Inport
  Trigger : TriggerPort  TriggerType=falling
  Light Sensor Switch OFF : S-Function  FunctionName=sfun_light_sw  Parameters=-1,ip,sw  EnableBusSupport=off  mask(Light Sensor ON/OFF Switch){ip=S3, sw=OFF}
      mask prompts: ip "port:"; sw "switch"
      mask help: LEGO Mindstorms NXT Light Sensor switch.
      mask init:
      | [data, map]=imread('LIGHT_SENSOR.gif');
      | pic=ind2rgb(data,map);
      mask TypeOptions ip: S1 | S2 | S3 | S4
      mask TypeOptions sw: ON | OFF
      mask Display:
      | image(pic)
      | color('red')
      | fprintf('%s, %s',ip,sw)
  Out1 : Outport
  wires:
  In1/1 -> Out1/1

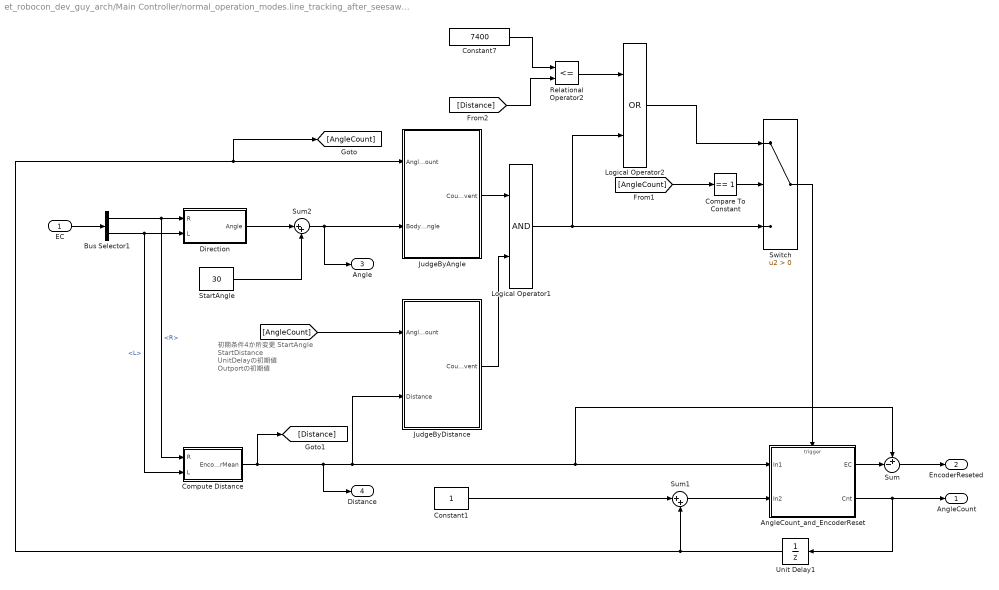
== system et_robocon_dev_guy_arch/Main Controller/normal_operation_modes.line_tracking_after_seesaw/line_tracking_mode.Track.analyzeEncoders/AngleCounter ==
  note: 初期条件4か所変更
      | StartAngle
      | StartDistance
      | UnitDelayの初期値
      | Outportの初期値
  EC : Inport
  AngleCount_and_EncoderReset : Subsystem  TreatAsAtomicUnit=on
  Bus Selector1 : BusSelector  OutputSignals=R,L
  Compare To Constant : simulink/Logic and Bit Operations/Compare To Constant  relop===  const=1  OutDataTypeStr=boolean
  Compute Distance : Subsystem
  Constant1 : Constant  OutDataTypeStr=uint8
  Constant7 : Constant  Value=7400  OutDataTypeStr=int32
  Direction : Subsystem
  JudgeByAngle : Subsystem
  JudgeByDistance : Subsystem
  Logical Operator1 : Logic  AllPortsSameDT=off  OutDataTypeStr=boolean
  Logical Operator2 : Logic  Operator=OR  AllPortsSameDT=off  OutDataTypeStr=boolean
  Relational Operator2 : RelationalOperator  Operator=<=  OutDataTypeStr=boolean
  StartAngle : Constant  Value=30  OutDataTypeStr=int16
  Sum : Sum  Inputs=+-|
  Sum1 : Sum  Inputs=|++  AccumDataTypeStr=uint8
  Sum2 : Sum  Inputs=|++
  Switch : Switch  Criteria=u2 > Threshold
  Unit Delay1 : UnitDelay  InitialCondition=1  SampleTime=-1
  AngleCount : Outport
  EncoderReseted : Outport  Port=2
  Angle : Outport  Port=3
  Distance : Outport  Port=4
  wires:
  Sum2/1 -> JudgeByAngle/2(BodyAngle), Angle/1
  Sum1/1 -> AngleCount_and_EncoderReset/2(In2)
  Constant1/1 -> Sum1/1
  Unit Delay1/1 -> [AngleCount], JudgeByAngle/1(AngleCount), Sum1/2
  AngleCount_and_EncoderReset/2(Cnt) -> AngleCount/1, Unit Delay1/1
  Bus Selector1/1 -> Compute Distance/1(R), Direction/1(R)  "<R>"
  Bus Selector1/2 -> Compute Distance/2(L), Direction/2(L)  "<L>"
  EC/1 -> Bus Selector1/1
  AngleCount_and_EncoderReset/1(EC) -> Sum/2
  Sum/1 -> EncoderReseted/1
  Compute Distance/1(EncoderMean) -> [Distance], Distance/1, JudgeByDistance/2(Distance), Sum/1, AngleCount_and_EncoderReset/1(In1)
  [AngleCount] -> JudgeByDistance/1(AngleCount)
  JudgeByAngle/1(CountEvent) -> Logical Operator1/1
  JudgeByDistance/1(CountEvent) -> Logical Operator1/2
  Direction/1(Angle) -> Sum2/1
  StartAngle/1 -> Sum2/2
  Logical Operator1/1 -> Logical Operator2/2, Switch/3
  Switch/1 -> AngleCount_and_EncoderReset/Trigger
  Compare To Constant/1 -> Switch/2
  [AngleCount] -> Compare To Constant/1
  Logical Operator2/1 -> Switch/1
  Constant7/1 -> Relational Operator2/1
  Relational Operator2/1 -> Logical Operator2/1
  [Distance] -> Relational Operator2/2

== system et_robocon_dev_guy_arch/Main Controller/normal_operation_modes.line_tracking_after_seesaw/line_tracking_mode.Track.analyzeEncoders/Store x0 ==
  In1 : Inport
  In2 : Inport  Port=2
  Enable : EnablePort
  Out1 : Outport
  Out2 : Outport  Port=2
  wires:
  In1/1 -> Out1/1
  In2/1 -> Out2/1

== system et_robocon_dev_guy_arch/Main Controller/normal_operation_modes.line_tracking_after_seesaw/line_tracking_mode.Track.lineTracker/Handler ==
  steering : Inport
  fwd : Inport  Port=2
  Constant1 : Constant  Value=-1  OutDataTypeStr=int8
  Mux : Mux  Inputs=2
  Switch1 : Switch  OutDataTypeStr=single  RndMeth=Simplest
  rocket_start : Subsystem
  slow_start : Subsystem
  cmd : Outport
  wires:
  steering/1 -> Mux/2  "str"
  slow_start/1(fwd_slow) -> Switch1/1
  Mux/1 -> cmd/1
  fwd/1 -> rocket_start/1(fwd), slow_start/1(fwd)  "fwd"
  Constant1/1 -> Switch1/2
  rocket_start/1(fwd_slow) -> Switch1/3
  Switch1/1 -> Mux/1

== system et_robocon_dev_guy_arch/Main Controller/normal_operation_modes.line_tracking_after_seesaw/line_tracking_mode.Track.lineTracker/SwitchForFreeSteering ==
  note: Edge Change
      | -1: Run right edge
      | 1: Run left edge
  note: Target Value
  FlagSteering : Inport
  PID : Inport  Port=2  PortDimensions=5
  LightSens : Inport  Port=3
  Add : Sum  Inputs=+-  AccumDataTypeStr=single  OutDataTypeStr=single  RndMeth=Simplest
  AdjustForUnit : Gain  Gain=18.25  OutDataTypeStr=single  RndMeth=Simplest
  Constant2 : Constant  OutDataTypeStr=single  SampleTime=-1
  Constant6 : Constant  Value=0.5  OutDataTypeStr=single  SampleTime=-1
  DeleteDummyData : Selector  InputPortWidth=5  IndexOptions=Index vector (dialog)  Indices=1  OutputSizes=1
  Product1 : Product  OutDataTypeStr=single  RndMeth=Simplest
  Switch : Switch  Criteria=u2 > Threshold
  tmpController : Subsystem  TreatAsAtomicUnit=on  mask(tmp PID Controller){Ts_=ts2, SaturationMax=100, SaturationMin=-100}
      mask prompts: Ts_ "Sampling Time (Task Period)"; SaturationMax "Saturation Max Value of PID Ctrl"; SaturationMin "Saturation Min Value of PID"
      mask help:
      | Sampling Time: Task Period
      | P: Proportional Gain
      | I: Integral Gain
      | D: Derivative Gain
      | B: Back Gain for Integrator
      | Saturation Max Value of PID ctrl:
      |    Saturation Max Value of PID ctrl > Saturation Min Value of PID ctrl
      | Saturation Min Value of PID ctrl:
      |    Saturation Min Value of PID ctrl < Saturation Max Value of PID ctrl
      settings: RTWSystemCode=Inline
      mask Display: disp('PID')
  Steering : Outport
  wires:
  PID/1 -> tmpController/2(BD), DeleteDummyData/1
  Switch/1 -> Steering/1
  DeleteDummyData/1 -> Switch/1  "FreeSteering"
  FlagSteering/1 -> Switch/2
  Add/1 -> Product1/1
  LightSens/1 -> Add/1
  Constant6/1 -> Add/2
  Constant2/1 -> Product1/2
  Product1/1 -> tmpController/1(Error)  "Diff_Between_Target_and_Value"
  tmpController/1(Target_deg) -> AdjustForUnit/1
  AdjustForUnit/1 -> Switch/3  "LintTraceSteering"

== system et_robocon_dev_guy_arch/Main Controller/normal_operation_modes.line_tracking_after_seesaw/line_tracking_mode.Track.processLight/OFF2ON ==
  In1 : Inport
  Trigger : TriggerPort
  Light Sensor Switch ON : S-Function  FunctionName=sfun_light_sw  Parameters=-1,ip,sw  EnableBusSupport=off  mask(Light Sensor ON/OFF Switch){ip=S3, sw=ON}
      mask prompts: ip "port:"; sw "switch"
      mask help: LEGO Mindstorms NXT Light Sensor switch.
      mask init:
      | [data, map]=imread('LIGHT_SENSOR.gif');
      | pic=ind2rgb(data,map);
      mask TypeOptions ip: S1 | S2 | S3 | S4
      mask TypeOptions sw: ON | OFF
      mask Display:
      | image(pic)
      | color('red')
      | fprintf('%s, %s',ip,sw)
  Out1 : Outport
  wires:
  In1/1 -> Out1/1

== system et_robocon_dev_guy_arch/Main Controller/normal_operation_modes.line_tracking_after_seesaw/line_tracking_mode.Track.processLight/ON2OFF ==
  In1 : Inport
  Trigger : TriggerPort  TriggerType=falling
  Light Sensor Switch OFF : S-Function  FunctionName=sfun_light_sw  Parameters=-1,ip,sw  EnableBusSupport=off  mask(Light Sensor ON/OFF Switch){ip=S3, sw=OFF}
      mask prompts: ip "port:"; sw "switch"
      mask help: LEGO Mindstorms NXT Light Sensor switch.
      mask init:
      | [data, map]=imread('LIGHT_SENSOR.gif');
      | pic=ind2rgb(data,map);
      mask TypeOptions ip: S1 | S2 | S3 | S4
      mask TypeOptions sw: ON | OFF
      mask Display:
      | image(pic)
      | color('red')
      | fprintf('%s, %s',ip,sw)
  Out1 : Outport
  wires:
  In1/1 -> Out1/1
